simulink model "aula7"  (R2022a)
settings: Solver=VariableStepAuto  StartTime=0.0  StopTime=10.0  RelTol=1e-3
settings Model: Creator=a2103303  LastModifiedBy=a2103303

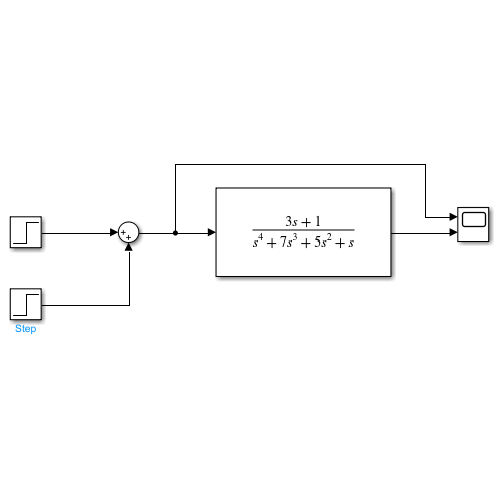
[thumbnail: Simulink's stored preview of the top-level diagram]
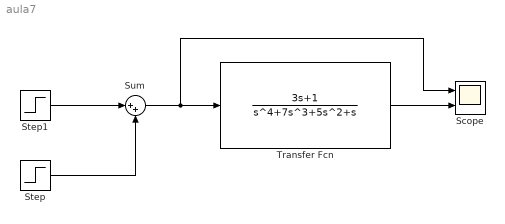
== system aula7 ==
  Scope : Scope  NumInputPorts=2
  Step : Step  SampleTime=0
  Step1 : Step  SampleTime=0
  Sum : Sum  Inputs=|++
  Transfer Fcn : TransferFcn  Numerator=[3 1]  Denominator=[1 7 5 1 0]
  wires:
  Step1/1 -> Sum/1
  Step/1 -> Sum/2
  Sum/1 -> Scope/1, Transfer Fcn/1
  Transfer Fcn/1 -> Scope/2
